simulink model "ex_410"  (R2018b)
settings: Solver=VariableStepAuto  StartTime=0.0  StopTime=3  RelTol=1e-3
settings Model: Creator=lenovo  LastModifiedBy=QJ-
settings DebuggingCC: LibraryContextMissingDiagnostic=none
settings SFSimCC: SimUseLocalCustomCode=off
settings RTWCC: RTWUseLocalCustomCode=off

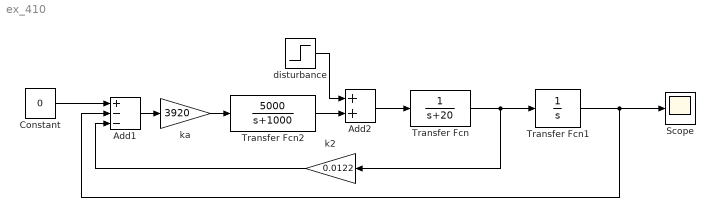
== system ex_410 ==
  Add1 : Sum  Inputs=+--
  Add2 : Sum
  Constant : Constant  Value=0
  Scope : Scope
  Transfer Fcn : TransferFcn  Denominator=[1 20]
  Transfer Fcn1 : TransferFcn  Denominator=[1 0]
  Transfer Fcn2 : TransferFcn  Numerator=[5000]  Denominator=[1 1000]
  disturbance : Step  SampleTime=1  mask(DiscretizedSource){}
      mask init:
      | %zoh
  k2 : Gain  Gain=0.0122
  ka : Gain  Gain=3920
  wires:
  Add2/1 -> Transfer Fcn/1
  disturbance/1 -> Add2/1
  Transfer Fcn2/1 -> Add2/2
  Transfer Fcn/1 -> k2/1, Transfer Fcn1/1
  Constant/1 -> Add1/1
  Transfer Fcn1/1 -> Add1/2, Scope/1
  ka/1 -> Transfer Fcn2/1
  k2/1 -> Add1/3
  Add1/1 -> ka/1
